simulink model "MotorModel"  (R2018a)
settings: Solver=VariableStepAuto  StartTime=0.0  StopTime=10  FixedStep=0.005  RelTol=1e-3
libraries: simulink x3
settings Model: Creator=Ammar Issa  LastModifiedBy=Ammar Issa

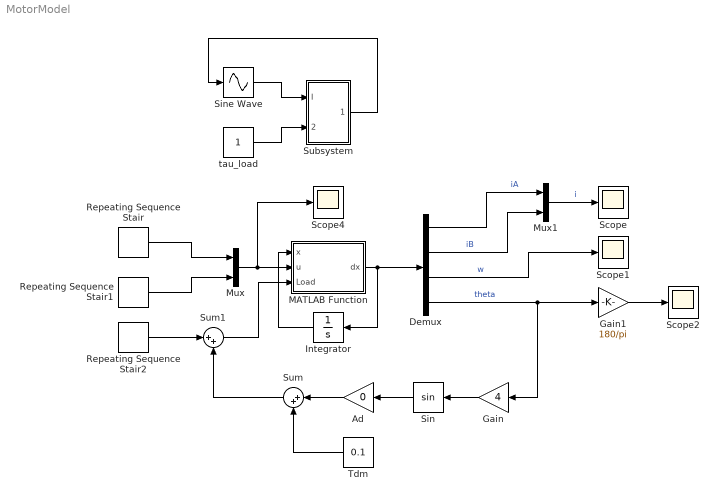
== system MotorModel ==
  Ad : Gain  Gain=0
  Demux : Demux
  Gain : Gain  Gain=4
  Gain1 : Gain  Gain=180/pi
  Integrator : Integrator  InitialCondition=[0; 0; 0; 0]
  MATLAB Function : MATLAB Function  TreatAsAtomicUnit=on
  Mux : Mux  Inputs=2
  Mux1 : Mux  Inputs=2
  Repeating Sequence Stair : simulink/Sources/Repeating Sequence Stair  OutValues=[1 0 -1 0].'  tsamp=0.05  OutMin=[]  OutMax=[]  OutDataTypeStr=double  OutputDataTypeScalingMode=double  OutDataType=fixdt(0,8)  ConRadixGroup=Best Precision: Vector-wise  OutScaling=2^-12
  Repeating Sequence Stair1 : simulink/Sources/Repeating Sequence Stair  OutValues=[0 1 0 -1].'  tsamp=0.05  OutMin=[]  OutMax=[]  OutDataTypeStr=double  OutputDataTypeScalingMode=double  OutDataType=fixdt(0,8)  ConRadixGroup=Best Precision: Vector-wise  OutScaling=2^-12
  Repeating Sequence Stair2 : simulink/Sources/Repeating Sequence Stair  OutValues=[0 1 0 -1].'  tsamp=0.5  OutMin=[]  OutMax=[]  OutDataTypeStr=double  OutputDataTypeScalingMode=double  OutDataType=fixdt(0,8)  ConRadixGroup=Best Precision: Vector-wise  OutScaling=2^-12
  Scope{,1..2,4} (4 alike) : Scope
  Sin : Trigonometry
  Sine Wave : Sin  TimeSource=Use external signal  Amplitude=2.8  SampleTime=0
  Subsystem : Subsystem
  Sum : Sum  Inputs=|++
  Sum1 : Sum  Inputs=|++
  Tdm : Constant  Value=0.1
  tau_load : Constant
  wires:
  Sine Wave/1 -> Subsystem/1(I)
  tau_load/1 -> Subsystem/2(Load)
  Subsystem/1(theta) -> Sine Wave/1
  MATLAB Function/1(dx) -> Integrator/1, Demux/1
  Integrator/1 -> MATLAB Function/1(x)
  Mux/1 -> Scope4/1, MATLAB Function/2(u)
  Mux1/1 -> Scope/1  "i"
  Demux/3 -> Scope1/1  "w"
  Demux/4 -> Gain1/1, Gain/1  "theta"
  Demux/1 -> Mux1/1  "iA"
  Demux/2 -> Mux1/2  "iB"
  Repeating Sequence Stair1/1 -> Mux/2
  Repeating Sequence Stair/1 -> Mux/1
  Gain/1 -> Sin/1
  Sin/1 -> Ad/1
  Ad/1 -> Sum/1
  Tdm/1 -> Sum/2
  Repeating Sequence Stair2/1 -> Sum1/1
  Sum/1 -> Sum1/2
  Sum1/1 -> MATLAB Function/3(Load)
  Gain1/1 -> Scope2/1

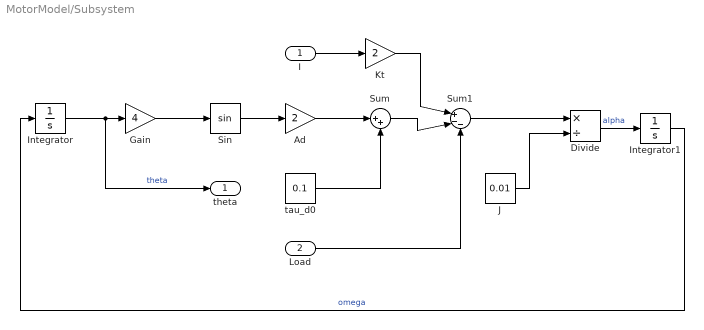
== system MotorModel/Subsystem ==
  I : Inport
  Load : Inport  Port=2
  Ad : Gain  Gain=2
  Divide : Product  Inputs=*/
  Gain : Gain  Gain=4
  Integrator : Integrator
  Integrator1 : Integrator
  J : Constant  Value=0.01
  Kt : Gain  Gain=2
  Sin : Trigonometry
  Sum : Sum  Inputs=|++
  Sum1 : Sum  Inputs=|+--
  tau_d0 : Constant  Value=0.1
  theta : Outport
  wires:
  Sum/1 -> Sum1/2
  Sum1/1 -> Divide/1
  Integrator1/1 -> Integrator/1  "omega"
  Integrator/1 -> theta/1, Gain/1  "theta"
  Sin/1 -> Ad/1
  Gain/1 -> Sin/1
  Kt/1 -> Sum1/1
  Ad/1 -> Sum/1
  tau_d0/1 -> Sum/2
  Load/1 -> Sum1/3
  J/1 -> Divide/2
  Divide/1 -> Integrator1/1  "alpha"
  I/1 -> Kt/1

== matlab function MotorModel/MATLAB Function ==
  data: x input; u input; dx output; Load input
function dx = fcn(x, u, Load)
    dx = zeros(4, 1);
    R = 5;
    L = 0.004;
    Km = 2;
    B = 0.05;
    J = 0.0001;
    Tdm = 0.1;
    p = 50;
    phi = 0;
    A = [-R/L, 0, Km/L, 0, 0;
         0, -R/L, -Km/L, 0, 0;
         -Km/J, Km/J, -B/J, -Tdm/J, -1/J];
    dx(1) = A(1, 1)*x(1) + A(1, 3)*x(3)*sin(p*x(4)) + u(1);
    dx(2) = A(2, 2)*x(2) + A(2, 3)*x(3)*cos(p*x(4)) + u(2);
    dx(3) = A(3, 1)*x(1)*sin(p*x(4)) + A(3, 2)*x(2)*cos(p*x(4)) + A(3, 3)*x(3) + A(3, 4)*sin(2*p*x(4) + phi) + A(3, 5)*Load;
    dx(4) = x(3);
end
